simulink model "HVACandHoodSystem"  (R2020b)
settings: Solver=VariableStepAuto  StartTime=0.0  StopTime=inf  RelTol=1e-3
libraries: simulink x2
settings Model: Creator=99003785  LastModifiedBy=99003785

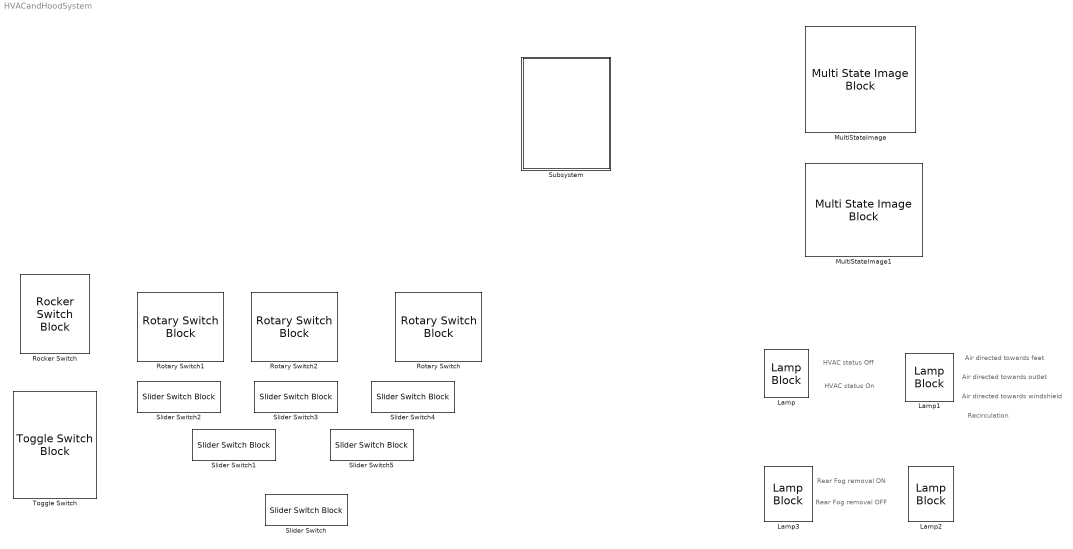
== system HVACandHoodSystem ==
  note: Rear Fog removal OFF
  note: Rear Fog removal ON
  note: Recirculation
  note: Air directed towards windshield
  note: Air directed towards outlet
  note: Air directed towards feet
  note: HVAC status Off
  note: HVAC status On
  Lamp{,1..3} (4 alike) : LampBlock
  MultiStateImage : MultiStateImageBlock
  MultiStateImage1 : MultiStateImageBlock
  Rocker Switch : RockerSwitchBlock
      settings: Values={{'On', 'Off'}, [1 0]}
  Rotary Switch : RotarySwitchBlock
      settings: Values={{'Off', 'Low', 'Medium', 'High'}, [0 1 2 3]}
  Rotary Switch1 : RotarySwitchBlock
      settings: Values={{'Off', 'Low', 'Medium', 'High'}, [0 1 2 3]}
  Rotary Switch2 : RotarySwitchBlock
      settings: Values={{'Off', 'AC', 'Heater', 'Air-Vent'}, [0 1 2 3]}
  Slider Switch{,1..5} (6 alike) : SliderSwitchBlock
      settings: Values={{'Off', 'On'}, [0 1]}
  Subsystem : Subsystem
  Toggle Switch : ToggleSwitchBlock
      settings: Values={{'Off', 'On'}, [0 1]}

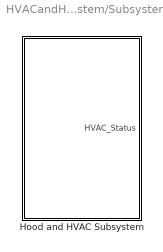
== system HVACandHoodSystem/Subsystem ==
  Hood and HVAC Subsystem : Subsystem  TreatAsAtomicUnit=on

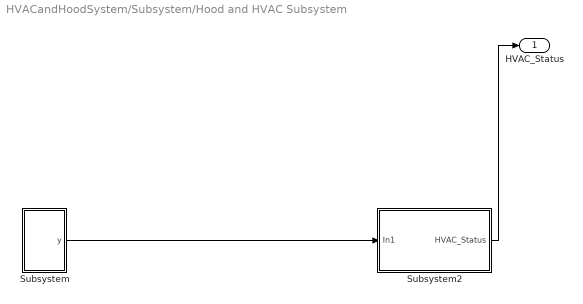
== system HVACandHoodSystem/Subsystem/Hood and HVAC Subsystem ==
  Subsystem : Subsystem
  Subsystem2 : Subsystem
  HVAC_Status : Outport
  wires:
  Subsystem/1(y) -> Subsystem2/1(In1)
  Subsystem2/1(HVAC_Status) -> HVAC_Status/1

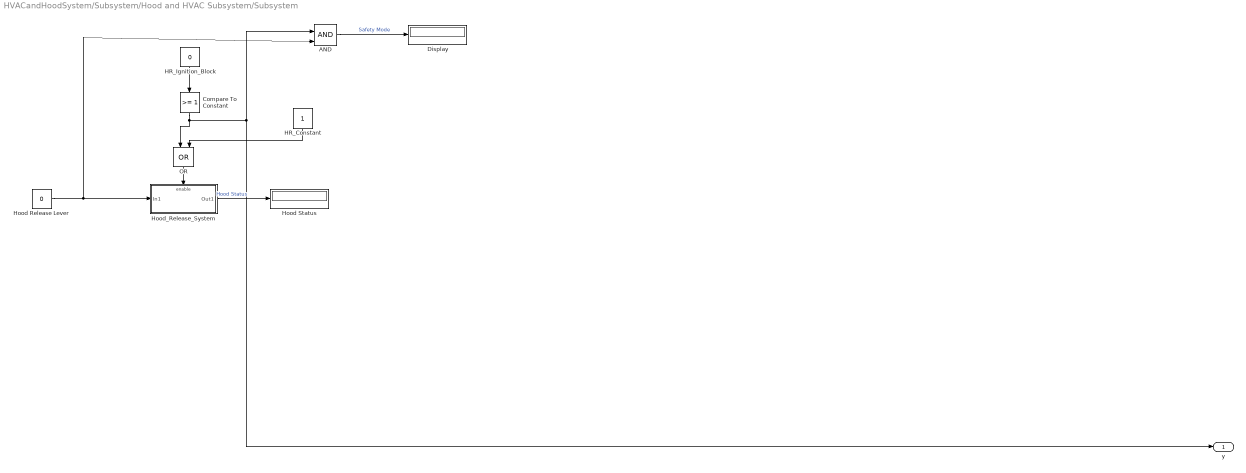
== system HVACandHoodSystem/Subsystem/Hood and HVAC Subsystem/Subsystem ==
  AND : Logic  IconShape=distinctive  AllPortsSameDT=off  OutDataTypeStr=boolean
  Compare To Constant : simulink/Logic and Bit Operations/Compare To Constant  relop=>=  const=1  OutDataTypeStr=boolean
  Display : Display
  HR_Constant : Constant
  HR_Ignition_Block : Constant  Value=0
  Hood Release Lever : Constant  Value=0
  Hood Status : Display
  Hood_Release_System : Subsystem  TreatAsAtomicUnit=on
  OR : Logic  Operator=OR  IconShape=distinctive  AllPortsSameDT=off  OutDataTypeStr=boolean
  y : Outport
  wires:
  OR/1 -> Hood_Release_System/Enable
  HR_Constant/1 -> OR/2
  Compare To Constant/1 -> y/1, AND/1, OR/1
  Hood Release Lever/1 -> AND/2, Hood_Release_System/1(In1)
  HR_Ignition_Block/1 -> Compare To Constant/1
  AND/1 -> Display/1  "Safety Mode"
  Hood_Release_System/1(Out1) -> Hood Status/1  "Hood Status"

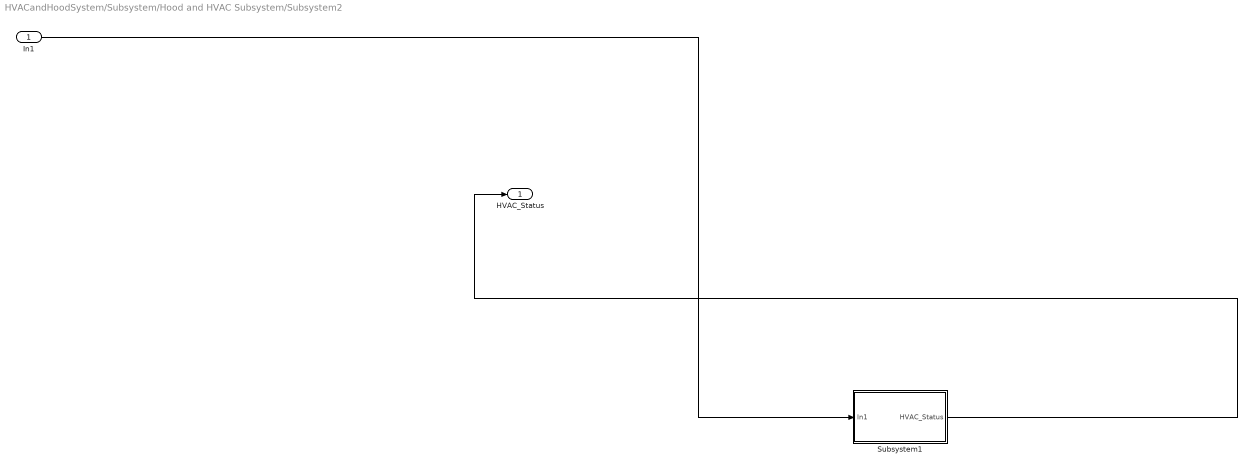
== system HVACandHoodSystem/Subsystem/Hood and HVAC Subsystem/Subsystem2 ==
  In1 : Inport
  Subsystem1 : Subsystem
  HVAC_Status : Outport
  wires:
  Subsystem1/1(HVAC_Status) -> HVAC_Status/1
  In1/1 -> Subsystem1/1(In1)

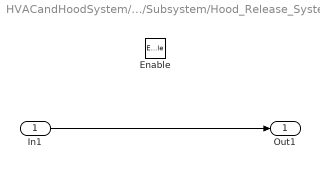
== system HVACandHoodSystem/Subsystem/Hood and HVAC Subsystem/Subsystem/Hood_Release_System ==
  In1 : Inport
  Enable : EnablePort
  Out1 : Outport  InitialOutput=0  VectorParamsAs1DForOutWhenUnconnected=off
  wires:
  In1/1 -> Out1/1

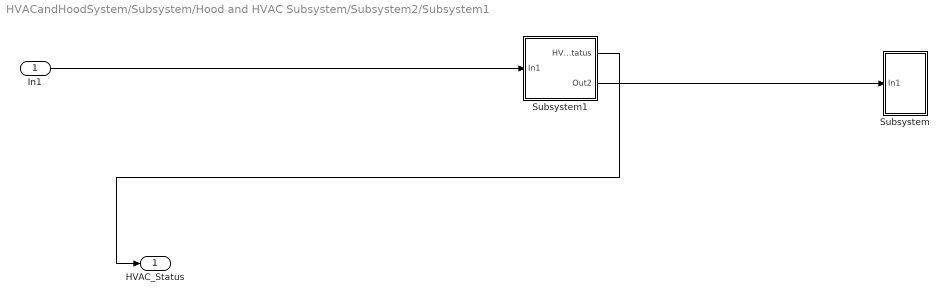
== system HVACandHoodSystem/Subsystem/Hood and HVAC Subsystem/Subsystem2/Subsystem1 ==
  In1 : Inport
  Subsystem : Subsystem
  Subsystem1 : Subsystem
  HVAC_Status : Outport
  wires:
  In1/1 -> Subsystem1/1(In1)
  Subsystem1/1(HVAC_Status) -> HVAC_Status/1
  Subsystem1/2(Out2) -> Subsystem/1(In1)

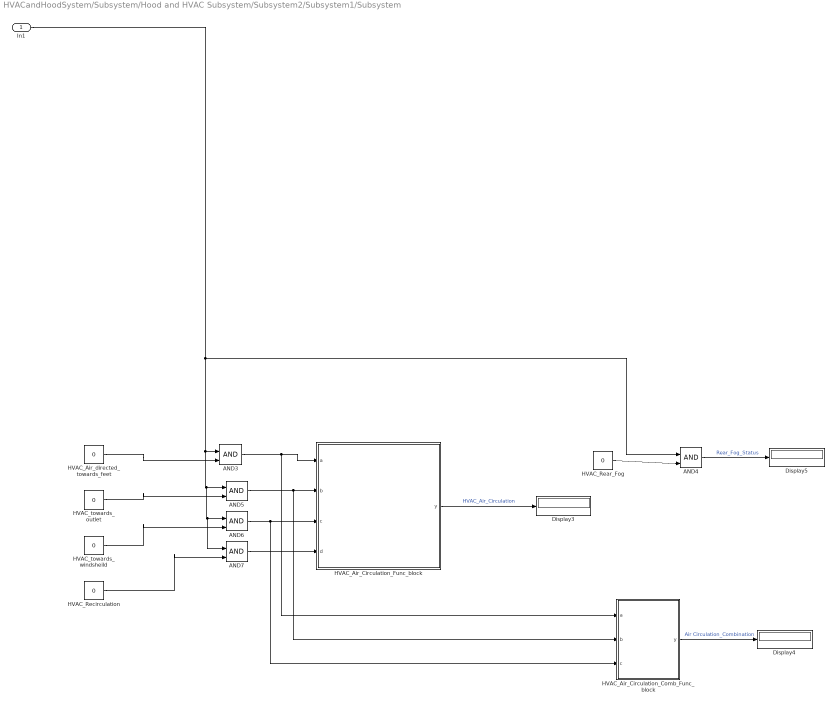
== system HVACandHoodSystem/Subsystem/Hood and HVAC Subsystem/Subsystem2/Subsystem1/Subsystem ==
  In1 : Inport
  AND{3..7} (5 alike) : Logic  IconShape=distinctive  AllPortsSameDT=off  OutDataTypeStr=boolean
  Display3 : Display
  Display4 : Display
  Display5 : Display
  HVAC_Air_Circulation_Comb_Func_block : MATLAB Function  TreatAsAtomicUnit=on
  HVAC_Air_Circulation_Func_block : MATLAB Function  TreatAsAtomicUnit=on
  HVAC_Air_directed_towards_feet : Constant  Value=0
  HVAC_Rear_Fog : Constant  Value=0
  HVAC_Recirculation : Constant  Value=0
  HVAC_towards_outlet : Constant  Value=0
  HVAC_towards_windsheild : Constant  Value=0
  wires:
  In1/1 -> AND4/1, AND7/1, AND6/1, AND5/1, AND3/1
  AND4/1 -> Display5/1  "Rear_Fog_Status"
  HVAC_Air_Circulation_Func_block/1(y) -> Display3/1  "HVAC_Air_Circulation"
  HVAC_Recirculation/1 -> AND7/2
  HVAC_towards_windsheild/1 -> AND6/2
  HVAC_Air_directed_towards_feet/1 -> AND3/2
  HVAC_Air_Circulation_Comb_Func_block/1(y) -> Display4/1  "Air Circulation_Combination"
  AND7/1 -> HVAC_Air_Circulation_Func_block/4(d)
  HVAC_towards_outlet/1 -> AND5/2
  AND6/1 -> HVAC_Air_Circulation_Comb_Func_block/3(c), HVAC_Air_Circulation_Func_block/3(c)
  AND3/1 -> HVAC_Air_Circulation_Comb_Func_block/1(a), HVAC_Air_Circulation_Func_block/1(a)
  HVAC_Rear_Fog/1 -> AND4/2
  AND5/1 -> HVAC_Air_Circulation_Comb_Func_block/2(b), HVAC_Air_Circulation_Func_block/2(b)

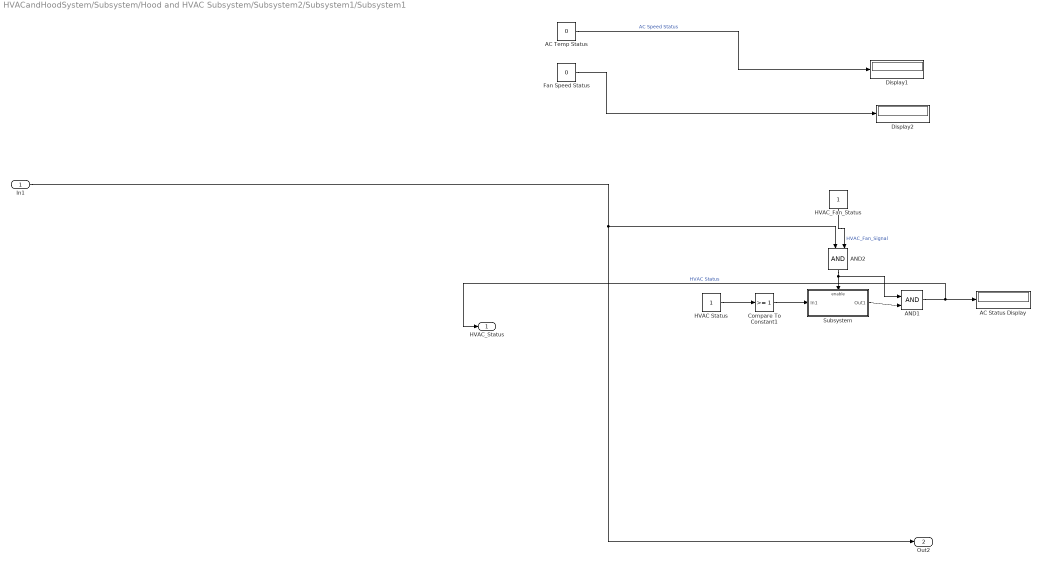
== system HVACandHoodSystem/Subsystem/Hood and HVAC Subsystem/Subsystem2/Subsystem1/Subsystem1 ==
  In1 : Inport
  AC Status Display : Display
  AC Temp Status : Constant  Value=0
  AND1 : Logic  IconShape=distinctive  AllPortsSameDT=off  OutDataTypeStr=boolean
  AND2 : Logic  IconShape=distinctive  AllPortsSameDT=off  OutDataTypeStr=boolean
  Compare To Constant1 : simulink/Logic and Bit Operations/Compare To Constant  relop=>=  const=1  OutDataTypeStr=boolean
  Display1 : Display
  Display2 : Display
  Fan Speed Status : Constant  Value=0
  HVAC Status : Constant
  HVAC_Fan_Status : Constant
  Subsystem : Subsystem
  HVAC_Status : Outport
  Out2 : Outport  Port=2
  wires:
  Fan Speed Status/1 -> Display2/1
  AND2/1 -> AND1/1, Subsystem/Enable
  AC Temp Status/1 -> Display1/1  "AC Speed Status"
  In1/1 -> Out2/1, AND2/1
  HVAC_Fan_Status/1 -> AND2/2  "HVAC_Fan_Signal"
  Compare To Constant1/1 -> Subsystem/1(In1)
  AND1/1 -> HVAC_Status/1, AC Status Display/1  "HVAC Status"
  Subsystem/1(Out1) -> AND1/2
  HVAC Status/1 -> Compare To Constant1/1

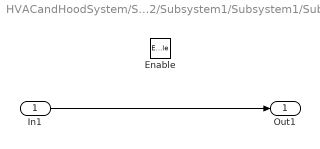
== system HVACandHoodSystem/Subsystem/Hood and HVAC Subsystem/Subsystem2/Subsystem1/Subsystem1/Subsystem ==
  In1 : Inport
  Enable : EnablePort
  Out1 : Outport
  wires:
  In1/1 -> Out1/1

== matlab function HVACandHoodSystem/Subsystem/Hood and HVAC Subsystem/Subsystem2/Subsystem1/Subsystem/HVAC_Air_Circulation_Comb_Func_block ==
  data: a input; b input; c input; y output
function y = fcn(a,b,c)
    if a==1&& b==1 && c==1
        y=1;
    elseif a==1 && b==1 && c==0
        y=2;
    elseif a==1 && b==0 && c==1
        y=3;
    elseif a==0 && b==1 && c==1
        y=4;
    else
        y=0;
    end

end

== matlab function HVACandHoodSystem/Subsystem/Hood and HVAC Subsystem/Subsystem2/Subsystem1/Subsystem/HVAC_Air_Circulation_Func_block ==
  data: a input; b input; y output; c input; d input
function y = fcn(a, b, c, d)
    if a==1 && b==0 && c==0 && d==0
        y=1;
    elseif a==0 && b==1 &&c==0 && d==0
        y=2;
    elseif a==0 && b==0 &&c==1 && d==0
        y=3;
    elseif a==0 && b==0 &&c==0 && d==1
        y=4;
    else
        y=0;
    end
    

end
